simulink model "PC_MSFS_STATION"  (R2021b)
settings: Solver=FixedStepAuto  StartTime=0.0  StopTime=2000  FixedStep=0.03  RelTol=1e-3
undefined symbols (not defined in the file): CONTROL, DiscIntNeverNeededParam, f, MODEL, MODEL_INI
libraries: instrumentlib x22, SimConnectToolbox x3, simulink x2
(part 1 of 2)
settings Model: Creator=Andreas  LastModifiedBy=ae-dagbeyibor3
settings SolverCC: AlgebraicLoopSolver=TrustRegion
settings DebuggingCC: InheritedTsInSrcMsg=none  SFMachineParentedDataDiag=warning

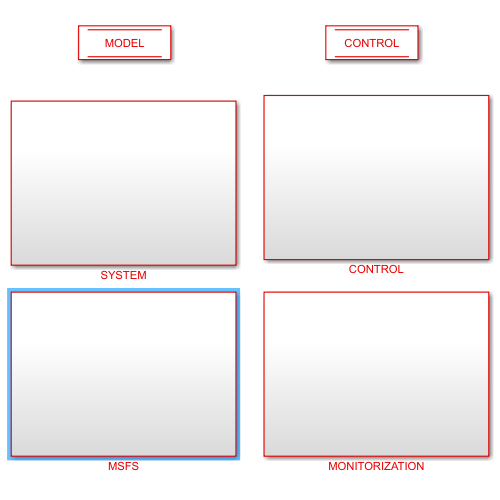
[thumbnail: Simulink's stored preview of the top-level diagram]
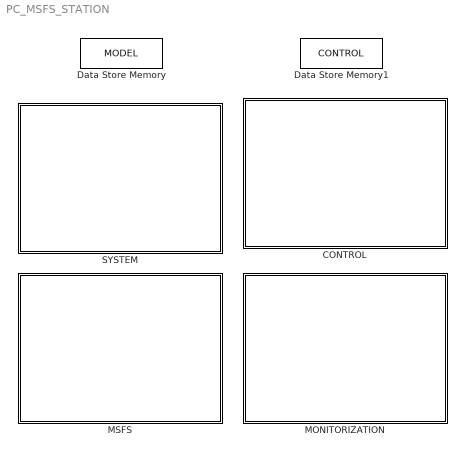
== system PC_MSFS_STATION ==
  CONTROL : Subsystem
  Data Store Memory : DataStoreMemory  DataStoreName=MODEL  ReadBeforeWriteMsg=warning  WriteAfterWriteMsg=warning  WriteAfterReadMsg=warning  InitialValue=MODEL_INI  ShowAdditionalParam=off  OutDataTypeStr=Bus: MODEL_Bus
  Data Store Memory1 : DataStoreMemory  DataStoreName=CONTROL  ReadBeforeWriteMsg=warning  WriteAfterWriteMsg=warning  WriteAfterReadMsg=warning  InitialValue=CONTROL_INI  ShowAdditionalParam=off  OutDataTypeStr=Bus: CONTROL_Bus
  MONITORIZATION : Subsystem
  MSFS : Subsystem
  SYSTEM : Subsystem

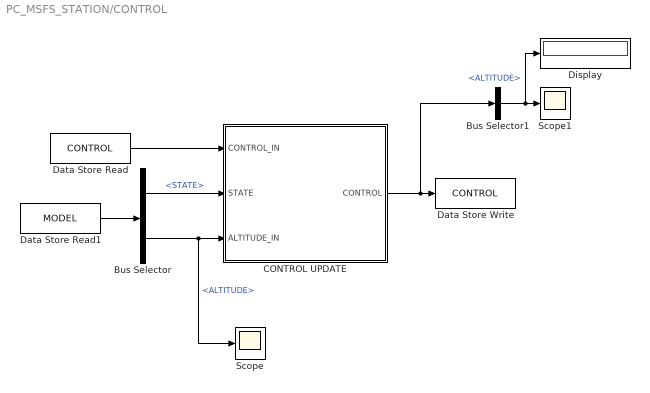
== system PC_MSFS_STATION/CONTROL ==
  Bus Selector : BusSelector  OutputSignals=STATE,INPUT.ALTITUDE
  Bus Selector1 : BusSelector  OutputSignals=PARAM.ALTITUDE
  CONTROL UPDATE : MATLAB Function  TreatAsAtomicUnit=on
  Data Store Read : DataStoreRead  DataStoreName=CONTROL  SampleTime=MODEL_INI.PARAM.SIM_SAMPLING_TIME  IndexOptions=Index vector (dialog)  Indices=1  OutputSizes=1
  Data Store Read1 : DataStoreRead  DataStoreName=MODEL  SampleTime=MODEL_INI.PARAM.SIM_SAMPLING_TIME  IndexOptions=Index vector (dialog)  Indices=1  OutputSizes=1
  Data Store Write : DataStoreWrite  DataStoreName=CONTROL  IndexOptions=Index vector (dialog)  Indices=1  OutputSizes=1
  Display : Display
  Scope : Scope
  Scope1 : Scope
  wires:
  Data Store Read/1 -> CONTROL UPDATE/1(CONTROL_IN)
  CONTROL UPDATE/1(CONTROL) -> Bus Selector1/1, Data Store Write/1
  Bus Selector/1 -> CONTROL UPDATE/2(STATE)  "<STATE>"
  Data Store Read1/1 -> Bus Selector/1
  Bus Selector/2 -> CONTROL UPDATE/3(ALTITUDE_IN), Scope/1  "<ALTITUDE>"
  Bus Selector1/1 -> Display/1, Scope1/1  "<ALTITUDE>"

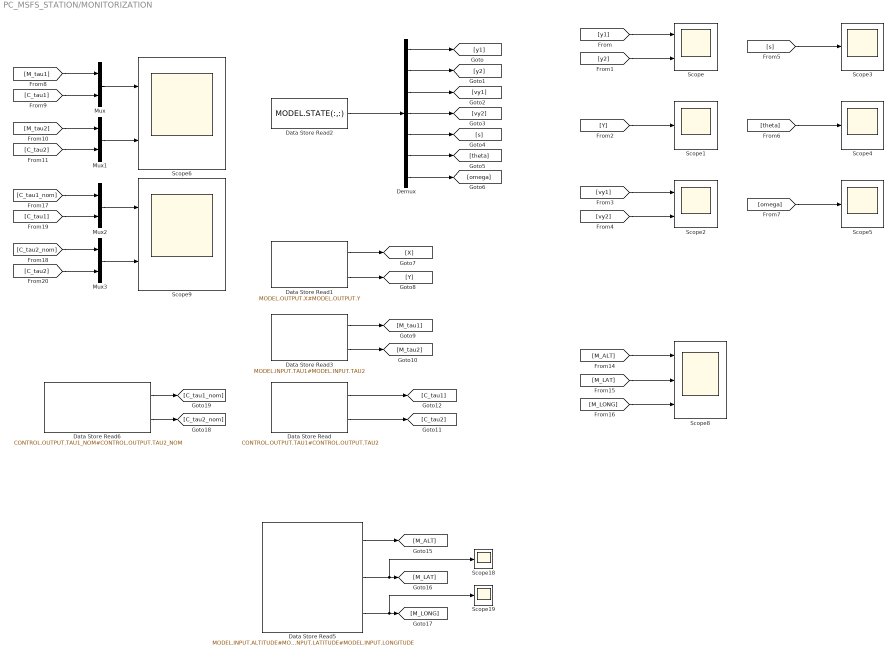
== system PC_MSFS_STATION/MONITORIZATION ==
  Data Store Read : DataStoreRead  DataStoreName=CONTROL  DataStoreElements=CONTROL.OUTPUT.TAU1#CONTROL.OUTPUT.TAU2  IndexOptions=Index vector (dialog)  Indices=1  OutputSizes=1
  Data Store Read1 : DataStoreRead  DataStoreName=MODEL  SampleTime=MODEL_INI.PARAM.SIM_SAMPLING_TIME  DataStoreElements=MODEL.OUTPUT.X#MODEL.OUTPUT.Y  IndexOptions=Index vector (dialog)  Indices=1  OutputSizes=1
  Data Store Read2 : DataStoreRead  DataStoreName=MODEL  SampleTime=MODEL_INI.PARAM.SIM_SAMPLING_TIME  DataStoreElements=MODEL.STATE(:,:)  IndexOptions=Index vector (dialog)  Indices=1  OutputSizes=1
  Data Store Read3 : DataStoreRead  DataStoreName=MODEL  SampleTime=MODEL_INI.PARAM.SIM_SAMPLING_TIME  DataStoreElements=MODEL.INPUT.TAU1#MODEL.INPUT.TAU2  IndexOptions=Index vector (dialog)  Indices=1  OutputSizes=1
  Data Store Read5 : DataStoreRead  DataStoreName=MODEL  SampleTime=MODEL_INI.PARAM.SIM_SAMPLING_TIME  DataStoreElements=MODEL.INPUT.ALTITUDE#MODEL.INPUT.LATITUDE#MODEL.INPUT.LONGITUDE  IndexOptions=Index vector (dialog)  Indices=1  OutputSizes=1
  Data Store Read6 : DataStoreRead  DataStoreName=CONTROL  DataStoreElements=CONTROL.OUTPUT.TAU1_NOM#CONTROL.OUTPUT.TAU2_NOM  IndexOptions=Index vector (dialog)  Indices=1  OutputSizes=1
  Demux : Demux  Outputs=7
  Mux{,1..3} (4 alike) : Mux  Inputs=2
  Scope{,2,6,9} (4 alike) : Scope  NumInputPorts=2
  Scope{1,3..5,18..19} (6 alike) : Scope
  Scope8 : Scope  NumInputPorts=3
  wires:
  Data Store Read2/1 -> Demux/1
  Demux/1 -> [y1]
  Demux/2 -> [y2]
  Demux/3 -> [vy1]
  Demux/4 -> [vy2]
  Demux/5 -> [s]
  Demux/6 -> [theta]
  Demux/7 -> [omega]
  [y1] -> Scope/1
  [y2] -> Scope/2
  Data Store Read1/1 -> [X]
  Data Store Read1/2 -> [Y]
  [Y] -> Scope1/1
  [vy2] -> Scope2/2
  [vy1] -> Scope2/1
  [s] -> Scope3/1
  [theta] -> Scope4/1
  [omega] -> Scope5/1
  Data Store Read3/1 -> [M_tau1]
  Data Store Read3/2 -> [M_tau2]
  Data Store Read/1 -> [C_tau1]
  Data Store Read/2 -> [C_tau2]
  Mux/1 -> Scope6/1
  Mux1/1 -> Scope6/2
  [M_tau1] -> Mux/1
  [M_tau2] -> Mux1/1
  [C_tau2] -> Mux1/2
  [C_tau1] -> Mux/2
  Data Store Read5/2 -> Scope18/1, [M_LAT]
  Data Store Read5/1 -> [M_ALT]
  Data Store Read5/3 -> Scope19/1, [M_LONG]
  [M_LAT] -> Scope8/2
  [M_ALT] -> Scope8/1
  [M_LONG] -> Scope8/3
  Data Store Read6/2 -> [C_tau2_nom]
  Data Store Read6/1 -> [C_tau1_nom]
  [C_tau1] -> Mux2/2
  [C_tau2] -> Mux3/2
  [C_tau2_nom] -> Mux3/1
  [C_tau1_nom] -> Mux2/1
  Mux3/1 -> Scope9/2
  Mux2/1 -> Scope9/1

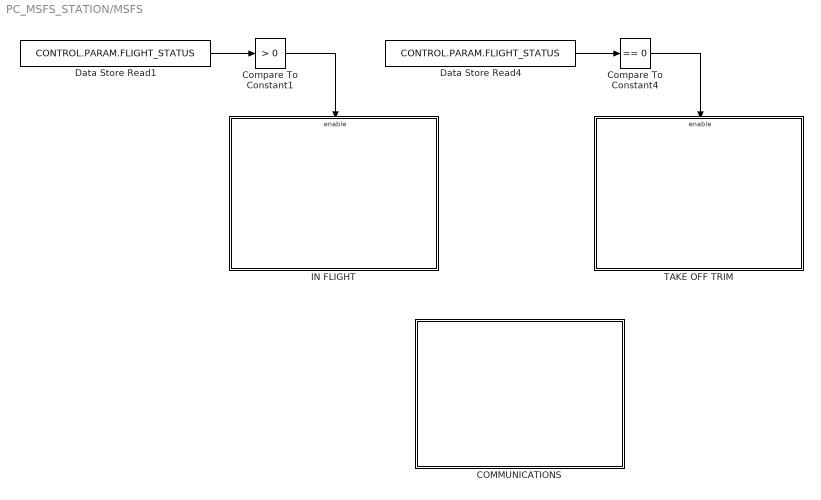
== system PC_MSFS_STATION/MSFS ==
  COMMUNICATIONS : Subsystem
  Compare To Constant1 : simulink/Logic and Bit Operations/Compare To Constant  relop=>  const=0  OutDataTypeStr=boolean
  Compare To Constant4 : simulink/Logic and Bit Operations/Compare To Constant  relop===  const=0  OutDataTypeStr=boolean
  Data Store Read1 : DataStoreRead  DataStoreName=CONTROL  DataStoreElements=CONTROL.PARAM.FLIGHT_STATUS  IndexOptions=Index vector (dialog)  Indices=1  OutputSizes=1
  Data Store Read4 : DataStoreRead  DataStoreName=CONTROL  DataStoreElements=CONTROL.PARAM.FLIGHT_STATUS  IndexOptions=Index vector (dialog)  Indices=1  OutputSizes=1
  IN FLIGHT : Subsystem
  TAKE OFF TRIM : Subsystem
  wires:
  Data Store Read1/1 -> Compare To Constant1/1
  Data Store Read4/1 -> Compare To Constant4/1
  Compare To Constant4/1 -> TAKE OFF TRIM/Enable
  Compare To Constant1/1 -> IN FLIGHT/Enable

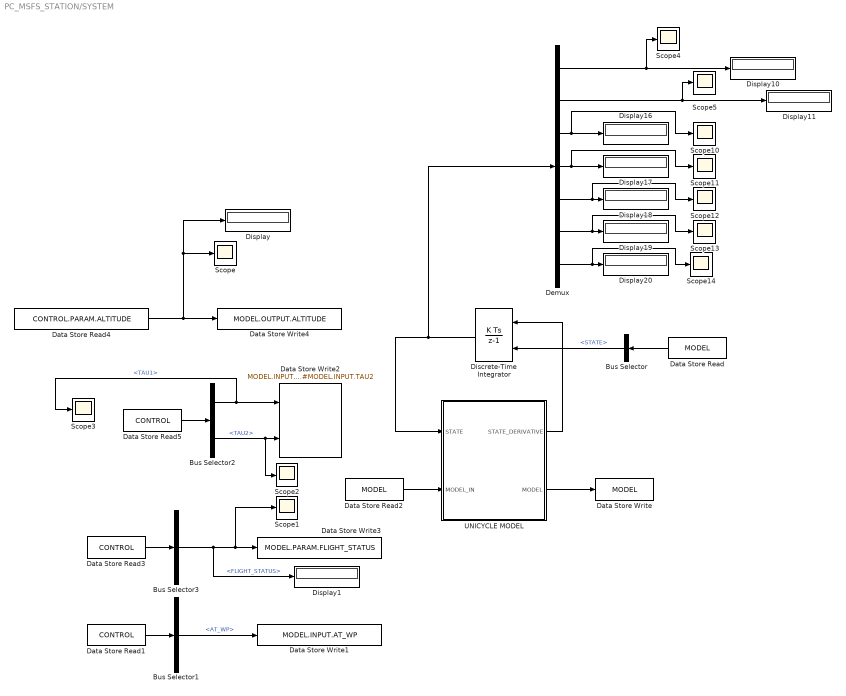
== system PC_MSFS_STATION/SYSTEM ==
  Bus Selector : BusSelector  OutputSignals=STATE
  Bus Selector1 : BusSelector  OutputSignals=OUTPUT.AT_WP
  Bus Selector2 : BusSelector  OutputSignals=OUTPUT.TAU1,OUTPUT.TAU2
  Bus Selector3 : BusSelector  OutputSignals=PARAM.FLIGHT_STATUS
  Data Store Read : DataStoreRead  DataStoreName=MODEL  SampleTime=MODEL_INI.PARAM.SIM_SAMPLING_TIME  IndexOptions=Index vector (dialog)  Indices=1  OutputSizes=1
  Data Store Read1 : DataStoreRead  DataStoreName=CONTROL  IndexOptions=Index vector (dialog)  Indices=1  OutputSizes=1
  Data Store Read2 : DataStoreRead  DataStoreName=MODEL  SampleTime=MODEL_INI.PARAM.SIM_SAMPLING_TIME  IndexOptions=Index vector (dialog)  Indices=1  OutputSizes=1
  Data Store Read3 : DataStoreRead  DataStoreName=CONTROL  IndexOptions=Index vector (dialog)  Indices=1  OutputSizes=1
  Data Store Read4 : DataStoreRead  DataStoreName=CONTROL  DataStoreElements=CONTROL.PARAM.ALTITUDE  IndexOptions=Index vector (dialog)  Indices=1  OutputSizes=1
  Data Store Read5 : DataStoreRead  DataStoreName=CONTROL  IndexOptions=Index vector (dialog)  Indices=1  OutputSizes=1
  Data Store Write : DataStoreWrite  DataStoreName=MODEL  IndexOptions=Index vector (dialog)  Indices=1  OutputSizes=1
  Data Store Write1 : DataStoreWrite  DataStoreName=MODEL  DataStoreElements=MODEL.INPUT.AT_WP  IndexOptions=Index vector (dialog)  Indices=1  OutputSizes=1
  Data Store Write2 : DataStoreWrite  DataStoreName=MODEL  DataStoreElements=MODEL.INPUT.TAU1#MODEL.INPUT.TAU2  IndexOptions=Index vector (dialog)  Indices=1  OutputSizes=1
  Data Store Write3 : DataStoreWrite  DataStoreName=MODEL  DataStoreElements=MODEL.PARAM.FLIGHT_STATUS  IndexOptions=Index vector (dialog)  Indices=1  OutputSizes=1
  Data Store Write4 : DataStoreWrite  DataStoreName=MODEL  DataStoreElements=MODEL.OUTPUT.ALTITUDE  IndexOptions=Index vector (dialog)  Indices=1  OutputSizes=1
  Demux : Demux  Outputs=7
  Discrete-Time Integrator : DiscreteIntegrator  InitialConditionSource=external  SampleTime=-1  ICPrevOutput=DiscIntNeverNeededParam  ICPrevScaledInput=DiscIntNeverNeededParam
  Display{,1,10..11,16..20} (9 alike) : Display
  Scope{,1..5,10..14} (11 alike) : Scope
  UNICYCLE MODEL : MATLAB Function  TreatAsAtomicUnit=on
  wires:
  Discrete-Time Integrator/1 -> Demux/1, UNICYCLE MODEL/1(STATE)
  UNICYCLE MODEL/1(STATE_DERIVATIVE) -> Discrete-Time Integrator/1
  Bus Selector/1 -> Discrete-Time Integrator/2  "<STATE>"
  Data Store Read/1 -> Bus Selector/1
  Data Store Read2/1 -> UNICYCLE MODEL/2(MODEL_IN)
  UNICYCLE MODEL/2(MODEL) -> Data Store Write/1
  Bus Selector2/2 -> Scope2/1, Data Store Write2/2  "<TAU2>"
  Bus Selector2/1 -> Scope3/1, Data Store Write2/1  "<TAU1>"
  Data Store Read5/1 -> Bus Selector2/1
  Data Store Read3/1 -> Bus Selector3/1
  Bus Selector3/1 -> Display1/1, Data Store Write3/1, Scope1/1  "<FLIGHT_STATUS>"
  Data Store Read4/1 -> Display/1, Scope/1, Data Store Write4/1
  Bus Selector1/1 -> Data Store Write1/1  "<AT_WP>"
  Data Store Read1/1 -> Bus Selector1/1
  Demux/1 -> Scope4/1, Display10/1
  Demux/2 -> Scope5/1, Display11/1
  Demux/6 -> Scope13/1, Display19/1
  Demux/3 -> Scope10/1, Display16/1
  Demux/4 -> Scope11/1, Display17/1
  Demux/5 -> Scope12/1, Display18/1
  Demux/7 -> Scope14/1, Display20/1

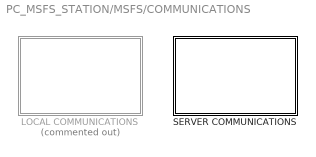
== system PC_MSFS_STATION/MSFS/COMMUNICATIONS ==
  LOCAL COMMUNICATIONS : Subsystem  Commented=on
  SERVER COMMUNICATIONS : Subsystem

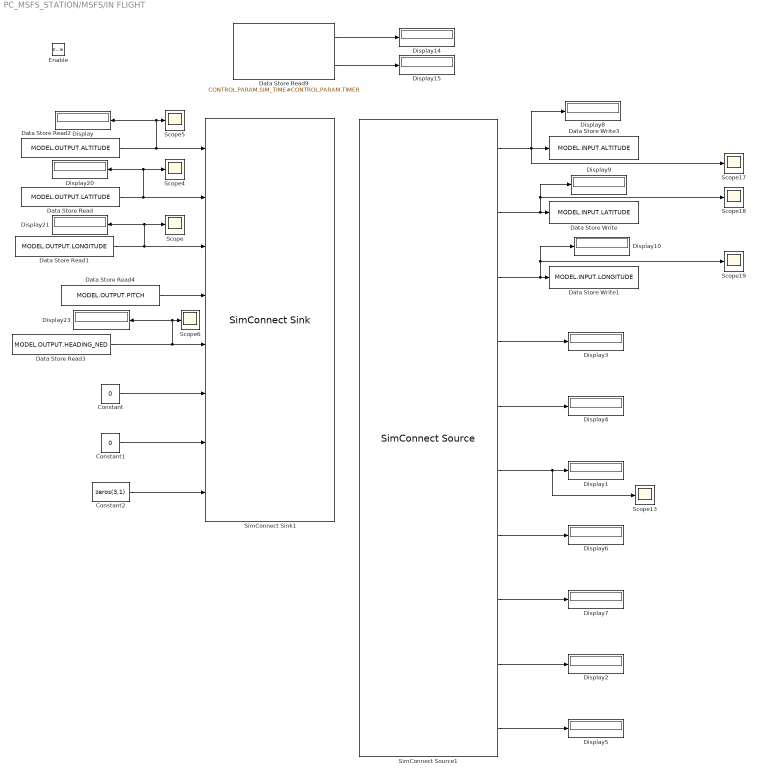
== system PC_MSFS_STATION/MSFS/IN FLIGHT ==
  Enable : EnablePort
  Constant : Constant  Value=0  SampleTime=-1
  Constant1 : Constant  Value=0  SampleTime=-1
  Constant2 : Constant  Value=zeros(3,1)  SampleTime=-1
  Data Store Read : DataStoreRead  DataStoreName=MODEL  DataStoreElements=MODEL.OUTPUT.LATITUDE  IndexOptions=Index vector (dialog)  Indices=1  OutputSizes=1
  Data Store Read1 : DataStoreRead  DataStoreName=MODEL  DataStoreElements=MODEL.OUTPUT.LONGITUDE  IndexOptions=Index vector (dialog)  Indices=1  OutputSizes=1
  Data Store Read2 : DataStoreRead  DataStoreName=MODEL  DataStoreElements=MODEL.OUTPUT.ALTITUDE  IndexOptions=Index vector (dialog)  Indices=1  OutputSizes=1
  Data Store Read3 : DataStoreRead  DataStoreName=MODEL  DataStoreElements=MODEL.OUTPUT.HEADING_NED  IndexOptions=Index vector (dialog)  Indices=1  OutputSizes=1
  Data Store Read4 : DataStoreRead  DataStoreName=MODEL  DataStoreElements=MODEL.OUTPUT.PITCH  IndexOptions=Index vector (dialog)  Indices=1  OutputSizes=1
  Data Store Read9 : DataStoreRead  DataStoreName=CONTROL  DataStoreElements=CONTROL.PARAM.SIM_TIME#CONTROL.PARAM.TIMER  IndexOptions=Index vector (dialog)  Indices=1  OutputSizes=1
  Data Store Write : DataStoreWrite  DataStoreName=MODEL  DataStoreElements=MODEL.INPUT.LATITUDE  IndexOptions=Index vector (dialog)  Indices=1  OutputSizes=1
  Data Store Write1 : DataStoreWrite  DataStoreName=MODEL  DataStoreElements=MODEL.INPUT.LONGITUDE  IndexOptions=Index vector (dialog)  Indices=1  OutputSizes=1
  Data Store Write3 : DataStoreWrite  DataStoreName=MODEL  DataStoreElements=MODEL.INPUT.ALTITUDE  IndexOptions=Index vector (dialog)  Indices=1  OutputSizes=1
  Display{,1..10,14..15,20..21,23} (16 alike) : Display
  Scope{,4..6,13,17..19} (8 alike) : Scope
  SimConnect Sink1 : SimConnectToolbox/SimConnect Sink  configurationIndex=0  connectionName=SimConnectSink  variables=|
      | PLANE ALTITUDE, FEET;
      | PLANE LATITUDE, RADIANS;
      | PLANE LONGITUDE, RADIANS;
      | PLANE PITCH DEGREES, RADIANS;
      | PLANE HEADING DEGREES TRUE, RADIANS;
      | PLANE BANK DEGREES, RADIANS;
      | AILERON POSITION, POSITION;
      | AILERON TRIM PCT, PERCENT;
      settings: SourceProductName=SimConnect Toolbox
      mask Display:
      | % This is a new mask on top of the base mask.
      | % Use "View base mask" link below to see the base mask.
      | %port_label('input', 1, 'Rudder Trim', 'texmode', 'on')
      | port_label('input', 1, 'PLANE ALTITUDE, FEET', 'texmode', 'on')
      | port_label('input', 2, 'PLANE LATITUDE, RADIANS', 'texmode', 'on')
      | port_label('input', 3, 'PLANE LONGITUDE, RADIANS', 'texmode', 'on')
      | port_label('input', 4, 'PITCH DEGREES, RADIANS', 'texmode', 'on')
      | port_label('input', 5, 'HEADING DEGREES TRUE, RADIANS', 'texmode', 'on')
      | port_label('input', 6, 'PLANE BANK DEGREES, RADIANS;', 'texmode', 'on')
      | port_label('input', 7, 'AILERON POSITION, POSITION', 'texmode', 'on')
      | port_label('input', 8, 'AILERON TRIM PCT, PERCENT OVER 100', 'texmode', 'on')
  SimConnect Source1 : SimConnectToolbox/SimConnect Source  configurationIndex=0  connectionName=SimConnectSource  variables=|
      | PLANE ALTITUDE, FEET;
      | PLANE LATITUDE, RADIANS;
      | PLANE LONGITUDE, RADIANS;
      | ROTATION VELOCITY BODY X, FEET PER SECOND;
      | PLANE PITCH DEGREES, RADIANS;
      | PLANE HEADING DEGREES TRUE, RADIANS;
      | PLANE HEADING DEGREES MAGNETIC, RADIANS;
      | PLANE HEADING DEGREES GYRO, DEGREES;
      | AILERON POSITION, POSITION;
      | AILERON TRIM PCT, PERCENT OVER 100;
      settings: SourceProductName=SimConnect Toolbox
      mask Display:
      | % This is a new mask on top of the base mask.
      | % Use "View base mask" link below to see the base mask.
      | % port_label('output', 1, 'g', 'texmode', 'on')
      | port_label('output', 1, 'PLANE ALTITUDE, FEET', 'texmode', 'on')
      | port_label('output', 2, 'PLANE LATITUDE, RADIANS', 'texmode', 'on')
      | port_label('output', 3, 'PLANE LONGITUDE, RADIANS', 'texmode', 'on')
      | port_label('output', 4, 'VELOCITY BODY X, FEET PER SECOND', 'texmode', 'on')
      | port_label('output', 5, 'PITCH DEGREES, RADIANS', 'texmode', 'on')
      | port_label('output', 6, 'HEADING DEGREES TRUE, RADIANS', 'texmode', 'on')
      | port_label('output', 7, 'HEADING DEGREES MAGNETIC, RADIANS', 'texmode', 'on')
      | port_label('output', 8, 'HEADING DEGREES GYRO, DEGREES', 'texmode', 'on')
      | port_label('output', 9, 'AILERON POSITION, POSITION', 'texmode', 'on')
      | port_label('output', 10, 'AILERON TRIM PCT, PERCENT OVER 100', 'texmode', 'on')
  wires:
  Constant2/1 -> SimConnect Sink1/8
  SimConnect Source1/9 -> Display2/1
  Constant/1 -> SimConnect Sink1/6
  Data Store Read1/1 -> Display21/1, Scope/1, SimConnect Sink1/3
  Constant1/1 -> SimConnect Sink1/7
  SimConnect Source1/5 -> Display4/1
  SimConnect Source1/3 -> Display10/1, Scope19/1, Data Store Write1/1
  SimConnect Source1/2 -> Display9/1, Scope18/1, Data Store Write/1
  SimConnect Source1/8 -> Display7/1
  SimConnect Source1/6 -> Scope13/1, Display1/1
  Data Store Read2/1 -> Display/1, Scope5/1, SimConnect Sink1/1
  Data Store Read/1 -> Display20/1, Scope4/1, SimConnect Sink1/2
  Data Store Read4/1 -> SimConnect Sink1/4
  SimConnect Source1/4 -> Display3/1
  SimConnect Source1/1 -> Data Store Write3/1, Display8/1, Scope17/1
  SimConnect Source1/7 -> Display6/1
  SimConnect Source1/10 -> Display5/1
  Data Store Read9/1 -> Display14/1
  Data Store Read9/2 -> Display15/1
  Data Store Read3/1 -> Display23/1, Scope6/1, SimConnect Sink1/5

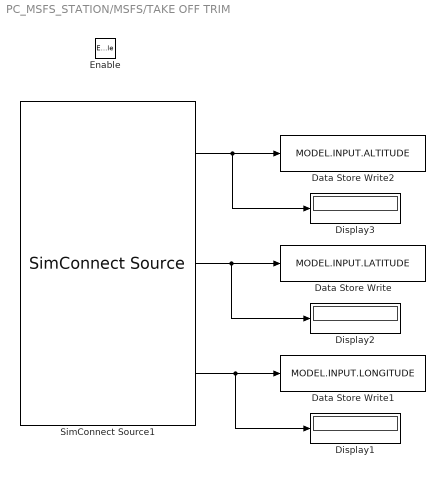
== system PC_MSFS_STATION/MSFS/TAKE OFF TRIM ==
  Enable : EnablePort
  Data Store Write : DataStoreWrite  DataStoreName=MODEL  DataStoreElements=MODEL.INPUT.LATITUDE  IndexOptions=Index vector (dialog)  Indices=1  OutputSizes=1
  Data Store Write1 : DataStoreWrite  DataStoreName=MODEL  DataStoreElements=MODEL.INPUT.LONGITUDE  IndexOptions=Index vector (dialog)  Indices=1  OutputSizes=1
  Data Store Write2 : DataStoreWrite  DataStoreName=MODEL  DataStoreElements=MODEL.INPUT.ALTITUDE  IndexOptions=Index vector (dialog)  Indices=1  OutputSizes=1
  Display1 : Display
  Display2 : Display
  Display3 : Display
  SimConnect Source1 : SimConnectToolbox/SimConnect Source  configurationIndex=0  connectionName=SimConnectSource  variables=|
      | PLANE ALTITUDE, FEET;
      | PLANE LATITUDE, RADIANS;
      | PLANE LONGITUDE, RADIANS;
      settings: SourceProductName=SimConnect Toolbox
      mask Display:
      | % This is a new mask on top of the base mask.
      | % Use "View base mask" link below to see the base mask.
      | % port_label('output', 1, 'g', 'texmode', 'on')
      | port_label('output', 1, 'PLANE ALTITUDE, FEET', 'texmode', 'on')
      | port_label('output', 2, 'PLANE LATITUDE, RADIANS', 'texmode', 'on')
      | port_label('output', 3, 'PLANE LONGITUDE, RADIANS', 'texmode', 'on')
  wires:
  SimConnect Source1/2 -> Data Store Write/1, Display2/1
  SimConnect Source1/1 -> Display3/1, Data Store Write2/1
  SimConnect Source1/3 -> Display1/1, Data Store Write1/1

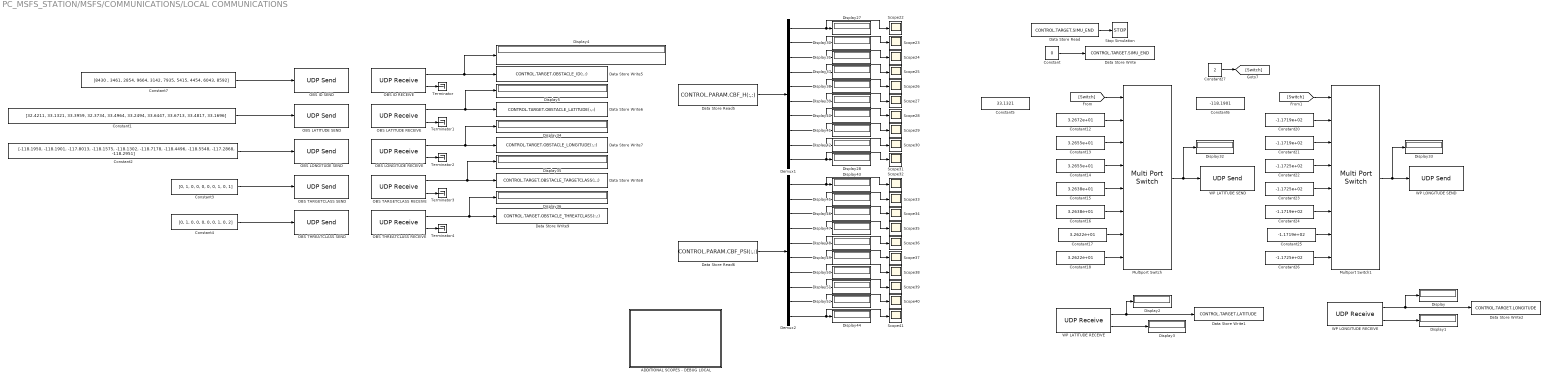
== system PC_MSFS_STATION/MSFS/COMMUNICATIONS/LOCAL COMMUNICATIONS ==
  ADDITIONAL SCOPES - DEBUG LOCAL : Subsystem
  Constant : Constant  Value=0  SampleTime=-1
  Constant1 : Constant  Value=[32.4211, 33.1321, 33.3959, 32.3734, 33.4964, 33.2494, 33.6447, 33.6713, 33.4817, 33.1696]  SampleTime=-1
  Constant12 : Constant  Value=3.2672e+01  SampleTime=0.03
  Constant13 : Constant  Value=3.2655e+01  SampleTime=0.03
  Constant14 : Constant  Value=3.2655e+01  SampleTime=0.03
  Constant15 : Constant  Value=3.2638e+01  SampleTime=0.03
  Constant16 : Constant  Value=3.2638e+01  SampleTime=0.03
  Constant17 : Constant  Value=3.2622e+01  SampleTime=0.03
  Constant18 : Constant  Value=3.2622e+01  SampleTime=0.03
  Constant2 : Constant  Value=[-118.1950, -118.1901, -117.8013, -118.1575, -118.1302, -118.7178, -118.4496, -118.5548, -117.2868, -118.2951]  SampleTime=-1
  Constant{20..21,24..25} (4 alike) : Constant  Value=-1.1719e+02  SampleTime=0.03
  Constant22 : Constant  Value=-1.1725e+02  SampleTime=0.03
  Constant23 : Constant  Value=-1.1725e+02  SampleTime=0.03
  Constant26 : Constant  Value=-1.1725e+02  SampleTime=0.03
  Constant27 : Constant  Value=2  SampleTime=-1
  Constant3 : Constant  Value=[0, 1, 0, 0, 0, 0, 0, 1, 0, 1]  SampleTime=-1
  Constant4 : Constant  Value=[0, 1, 0, 0, 0, 0, 0, 1, 0, 2]  SampleTime=-1
  Constant5 : Constant  Value=33.1321  SampleTime=0.03
  Constant6 : Constant  Value=-118.1901  SampleTime=0.03
  Constant7 : Constant  Value=[8430 , 3461, 2854, 9664, 3142, 7935, 5415, 4454, 6043, 8592]  SampleTime=-1
  Data Store Read : DataStoreRead  DataStoreName=CONTROL  DataStoreElements=CONTROL.TARGET.SIMU_END  IndexOptions=Index vector (dialog)  Indices=1  OutputSizes=1
  Data Store Read5 : DataStoreRead  DataStoreName=CONTROL  DataStoreElements=CONTROL.PARAM.CBF_H(:,:)  IndexOptions=Index vector (dialog)  Indices=1  OutputSizes=1
  Data Store Read6 : DataStoreRead  DataStoreName=CONTROL  DataStoreElements=CONTROL.PARAM.CBF_PSI(:,:)  IndexOptions=Index vector (dialog)  Indices=1  OutputSizes=1
  Data Store Write : DataStoreWrite  DataStoreName=CONTROL  DataStoreElements=CONTROL.TARGET.SIMU_END  IndexOptions=Index vector (dialog)  Indices=1  OutputSizes=1
  Data Store Write1 : DataStoreWrite  DataStoreName=CONTROL  DataStoreElements=CONTROL.TARGET.LATITUDE  IndexOptions=Index vector (dialog)  Indices=1  OutputSizes=1
  Data Store Write2 : DataStoreWrite  DataStoreName=CONTROL  DataStoreElements=CONTROL.TARGET.LONGITUDE  IndexOptions=Index vector (dialog)  Indices=1  OutputSizes=1
  Data Store Write5 : DataStoreWrite  DataStoreName=CONTROL  DataStoreElements=CONTROL.TARGET.OBSTACLE_ID(:,:)  IndexOptions=Index vector (dialog)  Indices=1  OutputSizes=1
  Data Store Write6 : DataStoreWrite  DataStoreName=CONTROL  DataStoreElements=CONTROL.TARGET.OBSTACLE_LATITUDE(:,:)  IndexOptions=Index vector (dialog)  Indices=1  OutputSizes=1
  Data Store Write7 : DataStoreWrite  DataStoreName=CONTROL  DataStoreElements=CONTROL.TARGET.OBSTACLE_LONGITUDE(:,:)  IndexOptions=Index vector (dialog)  Indices=1  OutputSizes=1
  Data Store Write8 : DataStoreWrite  DataStoreName=CONTROL  DataStoreElements=CONTROL.TARGET.OBSTACLE_TARGETCLASS(:,:)  IndexOptions=Index vector (dialog)  Indices=1  OutputSizes=1
  Data Store Write9 : DataStoreWrite  DataStoreName=CONTROL  DataStoreElements=CONTROL.TARGET.OBSTACLE_THREATCLASS(:,:)  IndexOptions=Index vector (dialog)  Indices=1  OutputSizes=1
  Demux1 : Demux  Outputs=10
  Demux2 : Demux  Outputs=10
  Display{,1..5,27..28,30..52} (31 alike) : Display
  Multiport Switch : MultiPortSwitch  Inputs=7
  Multiport Switch1 : MultiPortSwitch  Inputs=7
  OBS ID RECEIVE : instrumentlib/UDP Receive  Host=127.0.0.1  Port=8081  LocalPort=8082  EnablePortSharing=off  GetLatestData=off  DataSize="[10   1]"  DataType=double  ASCIIFormatting=%f,  Terminator=LF  ByteOrder=BigEndian  EnableBlockingMode=off  Timeout=10  SampleTime=-1  LocalAddress=127.0.0.1
  OBS ID SEND : instrumentlib/UDP Send  Host=127.0.0.1  Port=8082  LocalPort=8081  EnablePortSharing=off  ByteOrder=BigEndian  OutputDatagramPacketSize=512  EnableBlockingMode=on  LocalAddress=127.0.0.1
  OBS LATITUDE RECEIVE : instrumentlib/UDP Receive  Host=127.0.0.1  Port=8083  LocalPort=8084  EnablePortSharing=off  GetLatestData=off  DataSize="[10   1]"  DataType=double  ASCIIFormatting=%f,  Terminator=LF  ByteOrder=BigEndian  EnableBlockingMode=off  Timeout=10  SampleTime=-1  LocalAddress=127.0.0.1
  OBS LATITUDE SEND : instrumentlib/UDP Send  Host=127.0.0.1  Port=8084  LocalPort=8083  EnablePortSharing=off  ByteOrder=BigEndian  OutputDatagramPacketSize=512  EnableBlockingMode=on  LocalAddress=127.0.0.1
  OBS LONGITUDE RECEIVE : instrumentlib/UDP Receive  Host=127.0.0.1  Port=8085  LocalPort=8086  EnablePortSharing=off  GetLatestData=off  DataSize="[10   1]"  DataType=double  ASCIIFormatting=%f,  Terminator=LF  ByteOrder=BigEndian  EnableBlockingMode=off  Timeout=10  SampleTime=-1  LocalAddress=127.0.0.1
  OBS LONGITUDE SEND : instrumentlib/UDP Send  Host=127.0.0.1  Port=8086  LocalPort=8085  EnablePortSharing=off  ByteOrder=BigEndian  OutputDatagramPacketSize=512  EnableBlockingMode=on  LocalAddress=127.0.0.1
  OBS TARGETCLASS RECEIVE : instrumentlib/UDP Receive  Host=127.0.0.1  Port=7087  LocalPort=7088  EnablePortSharing=off  GetLatestData=off  DataSize="[10   1]"  DataType=double  ASCIIFormatting=%f,  Terminator=LF  ByteOrder=BigEndian  EnableBlockingMode=off  Timeout=10  SampleTime=-1  LocalAddress=127.0.0.1
  OBS TARGETCLASS SEND : instrumentlib/UDP Send  Host=127.0.0.1  Port=7088  LocalPort=7087  EnablePortSharing=off  ByteOrder=BigEndian  OutputDatagramPacketSize=512  EnableBlockingMode=on  LocalAddress=127.0.0.1
  OBS THREATCLASS RECEIVE : instrumentlib/UDP Receive  Host=127.0.0.1  Port=7089  LocalPort=7080  EnablePortSharing=off  GetLatestData=off  DataSize="[10   1]"  DataType=double  ASCIIFormatting=%f,  Terminator=LF  ByteOrder=BigEndian  EnableBlockingMode=off  Timeout=10  SampleTime=-1  LocalAddress=127.0.0.1
  OBS THREATCLASS SEND : instrumentlib/UDP Send  Host=127.0.0.1  Port=7080  LocalPort=7089  EnablePortSharing=off  ByteOrder=BigEndian  OutputDatagramPacketSize=512  EnableBlockingMode=on  LocalAddress=127.0.0.1
  Scope{22..41} (20 alike) : Scope
  Stop Simulation : Stop
  Terminator{,1..4} (5 alike) : Terminator
  WP LATITUDE RECEIVE : instrumentlib/UDP Receive  Host=127.0.0.1  Port=8087  LocalPort=8080  EnablePortSharing=off  GetLatestData=off  DataSize=[1 1]  DataType=double  ASCIIFormatting=%f,  Terminator=LF  ByteOrder=BigEndian  EnableBlockingMode=off  Timeout=10  SampleTime=-1  LocalAddress=127.0.0.1
  WP LATITUDE SEND : instrumentlib/UDP Send  Host=127.0.0.1  Port=8080  LocalPort=8087  EnablePortSharing=off  ByteOrder=BigEndian  OutputDatagramPacketSize=512  EnableBlockingMode=on  LocalAddress=127.0.0.1
  WP LONGITUDE RECEIVE : instrumentlib/UDP Receive  Host=127.0.0.1  Port=8089  LocalPort=8088  EnablePortSharing=off  GetLatestData=off  DataSize=[1 1]  DataType=double  ASCIIFormatting=%f,  Terminator=LF  ByteOrder=BigEndian  EnableBlockingMode=off  Timeout=10  SampleTime=-1  LocalAddress=127.0.0.1
  WP LONGITUDE SEND : instrumentlib/UDP Send  Host=127.0.0.1  Port=8088  LocalPort=8089  EnablePortSharing=off  ByteOrder=BigEndian  OutputDatagramPacketSize=512  EnableBlockingMode=on  LocalAddress=127.0.0.1
  wires:
  WP LATITUDE RECEIVE/2 -> Display3/1
  WP LATITUDE RECEIVE/1 -> Display2/1, Data Store Write1/1
  WP LONGITUDE RECEIVE/1 -> Data Store Write2/1, Display/1
  WP LONGITUDE RECEIVE/2 -> Display1/1
  Data Store Read/1 -> Stop Simulation/1
  Constant/1 -> Data Store Write/1
  [Switch] -> Multiport Switch/1
  Constant13/1 -> Multiport Switch/3
  Constant14/1 -> Multiport Switch/4
  Constant15/1 -> Multiport Switch/5
  Constant16/1 -> Multiport Switch/6
  Constant17/1 -> Multiport Switch/7
  Constant18/1 -> Multiport Switch/8
  Multiport Switch/1 -> WP LATITUDE SEND/1, Display32/1
  Multiport Switch1/1 -> WP LONGITUDE SEND/1, Display33/1
  Constant26/1 -> Multiport Switch1/8
  Constant25/1 -> Multiport Switch1/7
  Constant24/1 -> Multiport Switch1/6
  Constant23/1 -> Multiport Switch1/5
  Constant22/1 -> Multiport Switch1/4
  Constant21/1 -> Multiport Switch1/3
  [Switch] -> Multiport Switch1/1
  Constant27/1 -> [Switch]
  OBS ID RECEIVE/1 -> Data Store Write5/1, Display4/1
  OBS LATITUDE RECEIVE/1 -> Data Store Write6/1, Display5/1
  OBS LONGITUDE RECEIVE/1 -> Data Store Write7/1, Display34/1
  OBS TARGETCLASS RECEIVE/1 -> Display35/1, Data Store Write8/1
  OBS THREATCLASS RECEIVE/1 -> Display36/1, Data Store Write9/1
  OBS ID RECEIVE/2 -> Terminator/1
  OBS LATITUDE RECEIVE/2 -> Terminator1/1
  OBS LONGITUDE RECEIVE/2 -> Terminator2/1
  OBS TARGETCLASS RECEIVE/2 -> Terminator3/1
  OBS THREATCLASS RECEIVE/2 -> Terminator4/1
  Constant7/1 -> OBS ID SEND/1
  Constant1/1 -> OBS LATITUDE SEND/1
  Constant2/1 -> OBS LONGITUDE SEND/1
  Constant4/1 -> OBS THREATCLASS SEND/1
  Data Store Read5/1 -> Demux1/1
  Demux1/1 -> Scope22/1, Display27/1
  Demux1/2 -> Scope23/1, Display30/1
  Demux1/3 -> Scope24/1, Display31/1
  Demux1/4 -> Scope25/1, Display37/1
  Demux1/5 -> Scope26/1, Display38/1
  Demux1/6 -> Scope27/1, Display39/1
  Demux1/7 -> Scope28/1, Display40/1
  Demux1/8 -> Scope29/1, Display41/1
  Demux1/9 -> Scope30/1, Display42/1
  Demux1/10 -> Scope31/1, Display28/1
  Demux2/10 -> Display44/1, Scope41/1
  Demux2/9 -> Display52/1, Scope40/1
  Demux2/8 -> Display51/1, Scope39/1
  Demux2/7 -> Display50/1, Scope38/1
  Demux2/6 -> Display49/1, Scope37/1
  Demux2/5 -> Display48/1, Scope36/1
  Demux2/4 -> Display47/1, Scope35/1
  Demux2/3 -> Display46/1, Scope34/1
  Demux2/2 -> Display45/1, Scope33/1
  Demux2/1 -> Display43/1, Scope32/1
  Data Store Read6/1 -> Demux2/1
  Constant12/1 -> Multiport Switch/2
  Constant20/1 -> Multiport Switch1/2
  Constant3/1 -> OBS TARGETCLASS SEND/1

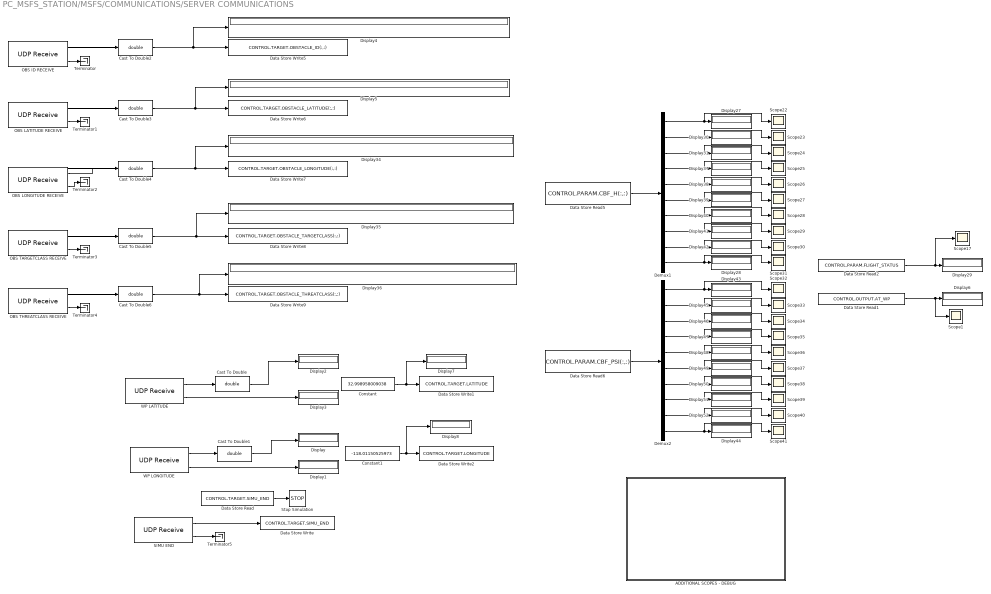
== system PC_MSFS_STATION/MSFS/COMMUNICATIONS/SERVER COMMUNICATIONS ==
  ADDITIONAL SCOPES - DEBUG : Subsystem
  Cast To Double{,1..6} (7 alike) : DataTypeConversion  OutDataTypeStr=double
  Constant : Constant  Value=32.998958009038  SampleTime=-1
  Constant1 : Constant  Value=-118.01150525973  SampleTime=-1
  Data Store Read : DataStoreRead  DataStoreName=CONTROL  DataStoreElements=CONTROL.TARGET.SIMU_END  IndexOptions=Index vector (dialog)  Indices=1  OutputSizes=1
  Data Store Read1 : DataStoreRead  DataStoreName=CONTROL  DataStoreElements=CONTROL.OUTPUT.AT_WP  IndexOptions=Index vector (dialog)  Indices=1  OutputSizes=1
  Data Store Read2 : DataStoreRead  DataStoreName=CONTROL  DataStoreElements=CONTROL.PARAM.FLIGHT_STATUS  IndexOptions=Index vector (dialog)  Indices=1  OutputSizes=1
  Data Store Read5 : DataStoreRead  DataStoreName=CONTROL  DataStoreElements=CONTROL.PARAM.CBF_H(:,:)  IndexOptions=Index vector (dialog)  Indices=1  OutputSizes=1
  Data Store Read6 : DataStoreRead  DataStoreName=CONTROL  DataStoreElements=CONTROL.PARAM.CBF_PSI(:,:)  IndexOptions=Index vector (dialog)  Indices=1  OutputSizes=1
  Data Store Write : DataStoreWrite  DataStoreName=CONTROL  DataStoreElements=CONTROL.TARGET.SIMU_END  IndexOptions=Index vector (dialog)  Indices=1  OutputSizes=1
  Data Store Write1 : DataStoreWrite  DataStoreName=CONTROL  DataStoreElements=CONTROL.TARGET.LATITUDE  IndexOptions=Index vector (dialog)  Indices=1  OutputSizes=1
  Data Store Write2 : DataStoreWrite  DataStoreName=CONTROL  DataStoreElements=CONTROL.TARGET.LONGITUDE  IndexOptions=Index vector (dialog)  Indices=1  OutputSizes=1
  Data Store Write5 : DataStoreWrite  DataStoreName=CONTROL  DataStoreElements=CONTROL.TARGET.OBSTACLE_ID(:,:)  IndexOptions=Index vector (dialog)  Indices=1  OutputSizes=1
  Data Store Write6 : DataStoreWrite  DataStoreName=CONTROL  DataStoreElements=CONTROL.TARGET.OBSTACLE_LATITUDE(:,:)  IndexOptions=Index vector (dialog)  Indices=1  OutputSizes=1
  Data Store Write7 : DataStoreWrite  DataStoreName=CONTROL  DataStoreElements=CONTROL.TARGET.OBSTACLE_LONGITUDE(:,:)  IndexOptions=Index vector (dialog)  Indices=1  OutputSizes=1
  Data Store Write8 : DataStoreWrite  DataStoreName=CONTROL  DataStoreElements=CONTROL.TARGET.OBSTACLE_TARGETCLASS(:,:)  IndexOptions=Index vector (dialog)  Indices=1  OutputSizes=1
  Data Store Write9 : DataStoreWrite  DataStoreName=CONTROL  DataStoreElements=CONTROL.TARGET.OBSTACLE_THREATCLASS(:,:)  IndexOptions=Index vector (dialog)  Indices=1  OutputSizes=1
  Demux1 : Demux  Outputs=10
  Demux2 : Demux  Outputs=10
  Display{,1..8,27..31,34..52} (33 alike) : Display
  OBS ID RECEIVE : instrumentlib/UDP Receive  Host=127.0.0.1  Port=8081  LocalPort=8082  EnablePortSharing=off  GetLatestData=off  DataSize="[10   1]"  DataType=double  ASCIIFormatting=%f,  Terminator=LF  ByteOrder=BigEndian  EnableBlockingMode=off  Timeout=10  SampleTime=-1  LocalAddress=127.0.0.1
  OBS LATITUDE RECEIVE : instrumentlib/UDP Receive  Host=127.0.0.1  Port=8083  LocalPort=8084  EnablePortSharing=off  GetLatestData=off  DataSize="[10   1]"  DataType=double  ASCIIFormatting=%f,  Terminator=LF  ByteOrder=BigEndian  EnableBlockingMode=off  Timeout=10  SampleTime=-1  LocalAddress=127.0.0.1
  OBS LONGITUDE RECEIVE : instrumentlib/UDP Receive  Host=127.0.0.1  Port=8085  LocalPort=8086  EnablePortSharing=off  GetLatestData=off  DataSize="[10   1]"  DataType=double  ASCIIFormatting=%f,  Terminator=LF  ByteOrder=BigEndian  EnableBlockingMode=off  Timeout=10  SampleTime=-1  LocalAddress=127.0.0.1
  OBS TARGETCLASS RECEIVE : instrumentlib/UDP Receive  Host=127.0.0.1  Port=7087  LocalPort=7088  EnablePortSharing=off  GetLatestData=off  DataSize="[10   1]"  DataType=double  ASCIIFormatting=%f,  Terminator=LF  ByteOrder=BigEndian  EnableBlockingMode=off  Timeout=10  SampleTime=-1  LocalAddress=127.0.0.1
  OBS THREATCLASS RECEIVE : instrumentlib/UDP Receive  Host=127.0.0.1  Port=7089  LocalPort=7080  EnablePortSharing=off  GetLatestData=off  DataSize="[10   1]"  DataType=double  ASCIIFormatting=%f,  Terminator=LF  ByteOrder=BigEndian  EnableBlockingMode=off  Timeout=10  SampleTime=-1  LocalAddress=127.0.0.1
  SIMU END : instrumentlib/UDP Receive  Host=127.0.0.1  Port=7086  LocalPort=7084  EnablePortSharing=off  GetLatestData=off  DataSize=[1 1]  DataType=double  ASCIIFormatting=%f,  Terminator=LF  ByteOrder=BigEndian  EnableBlockingMode=off  Timeout=10  SampleTime=-1  LocalAddress=127.0.0.1
  Scope{1,17,22..41} (22 alike) : Scope
  Stop Simulation : Stop
  Terminator{,1..5} (6 alike) : Terminator
  WP LATITUDE : instrumentlib/UDP Receive  Host=127.0.0.1  Port=8081  LocalPort=8080  EnablePortSharing=off  GetLatestData=off  DataSize=[1 1]  DataType=single  ASCIIFormatting=%f,  Terminator=LF  ByteOrder=BigEndian  EnableBlockingMode=off  Timeout=10  SampleTime=-1  LocalAddress=127.0.0.1
  WP LONGITUDE : instrumentlib/UDP Receive  Host=127.0.0.1  Port=8081  LocalPort=8088  EnablePortSharing=off  GetLatestData=off  DataSize=[1 1]  DataType=single  ASCIIFormatting=%f,  Terminator=LF  ByteOrder=BigEndian  EnableBlockingMode=off  Timeout=10  SampleTime=-1  LocalAddress=127.0.0.1
  wires:
  WP LONGITUDE/2 -> Display1/1
  Data Store Read1/1 -> Display6/1, Scope1/1
  Data Store Read2/1 -> Display29/1, Scope17/1
  WP LATITUDE/2 -> Display3/1
  WP LATITUDE/1 -> Cast To Double/1
  Cast To Double/1 -> Display2/1
  WP LONGITUDE/1 -> Cast To Double1/1
  Cast To Double1/1 -> Display/1
  Demux1/4 -> Scope25/1, Display37/1
  Demux1/2 -> Scope23/1, Display30/1
  Data Store Read6/1 -> Demux2/1
  Demux2/1 -> Display43/1, Scope32/1
  Demux2/3 -> Display46/1, Scope34/1
  Demux2/2 -> Display45/1, Scope33/1
  Demux2/7 -> Display50/1, Scope38/1
  Demux2/8 -> Display51/1, Scope39/1
  Demux2/9 -> Display52/1, Scope40/1
  Demux2/10 -> Display44/1, Scope41/1
  Demux2/6 -> Display49/1, Scope37/1
  Demux1/7 -> Scope28/1, Display40/1
  Demux2/4 -> Display47/1, Scope35/1
  Demux2/5 -> Display48/1, Scope36/1
  OBS ID RECEIVE/1 -> Cast To Double2/1
  Demux1/6 -> Scope27/1, Display39/1
  OBS LATITUDE RECEIVE/1 -> Cast To Double3/1
  Demux1/5 -> Scope26/1, Display38/1
  OBS THREATCLASS RECEIVE/1 -> Cast To Double6/1
  Demux1/9 -> Scope30/1, Display42/1
  OBS TARGETCLASS RECEIVE/2 -> Terminator3/1
  Demux1/8 -> Scope29/1, Display41/1
  OBS LONGITUDE RECEIVE/2 -> Terminator2/1
  OBS LATITUDE RECEIVE/2 -> Terminator1/1
  OBS ID RECEIVE/2 -> Terminator/1
  Demux1/1 -> Scope22/1, Display27/1
  OBS LONGITUDE RECEIVE/1 -> Cast To Double4/1
  Demux1/3 -> Scope24/1, Display31/1
  OBS TARGETCLASS RECEIVE/1 -> Cast To Double5/1
  OBS THREATCLASS RECEIVE/2 -> Terminator4/1
  Demux1/10 -> Scope31/1, Display28/1
  Data Store Read5/1 -> Demux1/1
  Cast To Double2/1 -> Data Store Write5/1, Display4/1
  Cast To Double3/1 -> Data Store Write6/1, Display5/1
  Cast To Double4/1 -> Data Store Write7/1, Display34/1
  Cast To Double5/1 -> Display35/1, Data Store Write8/1
  Cast To Double6/1 -> Display36/1, Data Store Write9/1
  Data Store Read/1 -> Stop Simulation/1
  SIMU END/2 -> Terminator5/1
  SIMU END/1 -> Data Store Write/1
  Constant/1 -> Display7/1, Data Store Write1/1
  Constant1/1 -> Display8/1, Data Store Write2/1

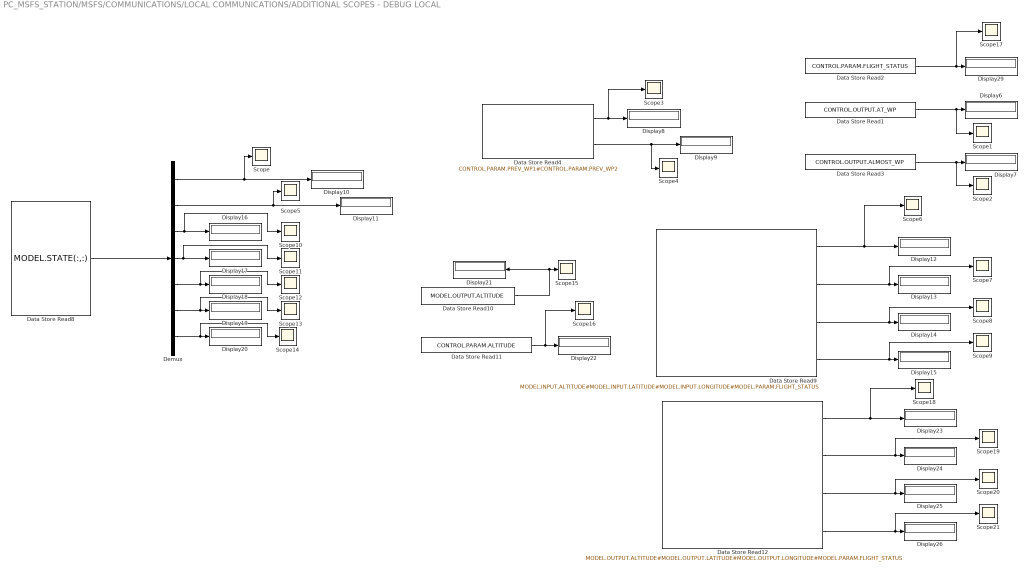
== system PC_MSFS_STATION/MSFS/COMMUNICATIONS/LOCAL COMMUNICATIONS/ADDITIONAL SCOPES - DEBUG LOCAL ==
  Data Store Read1 : DataStoreRead  DataStoreName=CONTROL  DataStoreElements=CONTROL.OUTPUT.AT_WP  IndexOptions=Index vector (dialog)  Indices=1  OutputSizes=1
  Data Store Read10 : DataStoreRead  DataStoreName=MODEL  DataStoreElements=MODEL.OUTPUT.ALTITUDE  IndexOptions=Index vector (dialog)  Indices=1  OutputSizes=1
  Data Store Read11 : DataStoreRead  DataStoreName=CONTROL  DataStoreElements=CONTROL.PARAM.ALTITUDE  IndexOptions=Index vector (dialog)  Indices=1  OutputSizes=1
  Data Store Read12 : DataStoreRead  DataStoreName=MODEL  DataStoreElements=MODEL.OUTPUT.ALTITUDE#MODEL.OUTPUT.LATITUDE#MODEL.OUTPUT.LONGITUDE#MODEL.PARAM.FLIGHT_STATUS  IndexOptions=Index vector (dialog)  Indices=1  OutputSizes=1
  Data Store Read2 : DataStoreRead  DataStoreName=CONTROL  DataStoreElements=CONTROL.PARAM.FLIGHT_STATUS  IndexOptions=Index vector (dialog)  Indices=1  OutputSizes=1
  Data Store Read3 : DataStoreRead  DataStoreName=CONTROL  DataStoreElements=CONTROL.OUTPUT.ALMOST_WP  IndexOptions=Index vector (dialog)  Indices=1  OutputSizes=1
  Data Store Read4 : DataStoreRead  DataStoreName=CONTROL  DataStoreElements=CONTROL.PARAM.PREV_WP1#CONTROL.PARAM.PREV_WP2  IndexOptions=Index vector (dialog)  Indices=1  OutputSizes=1
  Data Store Read8 : DataStoreRead  DataStoreName=MODEL  SampleTime=MODEL_INI.PARAM.SIM_SAMPLING_TIME  DataStoreElements=MODEL.STATE(:,:)  IndexOptions=Index vector (dialog)  Indices=1  OutputSizes=1
  Data Store Read9 : DataStoreRead  DataStoreName=MODEL  DataStoreElements=MODEL.INPUT.ALTITUDE#MODEL.INPUT.LATITUDE#MODEL.INPUT.LONGITUDE#MODEL.PARAM.FLIGHT_STATUS  IndexOptions=Index vector (dialog)  Indices=1  OutputSizes=1
  Demux : Demux  Outputs=7
  Display{6..26,29} (22 alike) : Display
  Scope{,1..21} (22 alike) : Scope
  wires:
  Demux/4 -> Scope11/1, Display17/1
  Data Store Read4/1 -> Scope3/1, Display8/1
  Data Store Read9/3 -> Scope8/1, Display14/1
  Data Store Read11/1 -> Scope16/1, Display22/1
  Data Store Read9/2 -> Scope7/1, Display13/1
  Demux/7 -> Scope14/1, Display20/1
  Data Store Read4/2 -> Scope4/1, Display9/1
  Data Store Read10/1 -> Display21/1, Scope15/1
  Data Store Read8/1 -> Demux/1
  Data Store Read2/1 -> Scope17/1, Display29/1
  Demux/5 -> Scope12/1, Display18/1
  Data Store Read12/2 -> Display24/1, Scope19/1
  Demux/3 -> Scope10/1, Display16/1
  Data Store Read9/4 -> Scope9/1, Display15/1
  Demux/6 -> Scope13/1, Display19/1
  Demux/2 -> Scope5/1, Display11/1
  Data Store Read9/1 -> Display12/1, Scope6/1
  Demux/1 -> Scope/1, Display10/1
  Data Store Read1/1 -> Scope1/1, Display6/1
  Data Store Read3/1 -> Scope2/1, Display7/1
  Data Store Read12/1 -> Scope18/1, Display23/1
  Data Store Read12/3 -> Display25/1, Scope20/1
  Data Store Read12/4 -> Display26/1, Scope21/1

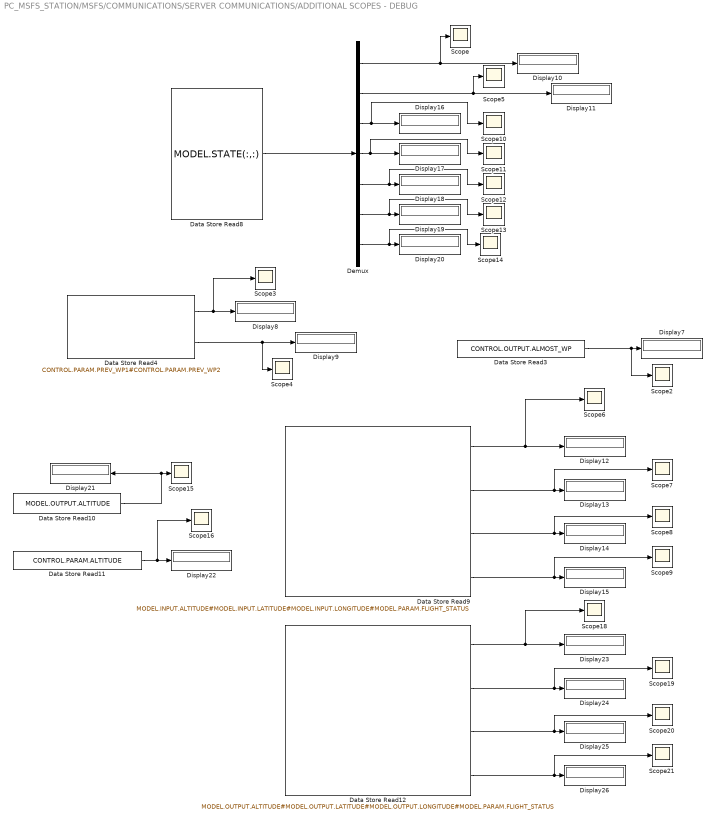
== system PC_MSFS_STATION/MSFS/COMMUNICATIONS/SERVER COMMUNICATIONS/ADDITIONAL SCOPES - DEBUG ==
  Data Store Read10 : DataStoreRead  DataStoreName=MODEL  DataStoreElements=MODEL.OUTPUT.ALTITUDE  IndexOptions=Index vector (dialog)  Indices=1  OutputSizes=1
  Data Store Read11 : DataStoreRead  DataStoreName=CONTROL  DataStoreElements=CONTROL.PARAM.ALTITUDE  IndexOptions=Index vector (dialog)  Indices=1  OutputSizes=1
  Data Store Read12 : DataStoreRead  DataStoreName=MODEL  DataStoreElements=MODEL.OUTPUT.ALTITUDE#MODEL.OUTPUT.LATITUDE#MODEL.OUTPUT.LONGITUDE#MODEL.PARAM.FLIGHT_STATUS  IndexOptions=Index vector (dialog)  Indices=1  OutputSizes=1
  Data Store Read3 : DataStoreRead  DataStoreName=CONTROL  DataStoreElements=CONTROL.OUTPUT.ALMOST_WP  IndexOptions=Index vector (dialog)  Indices=1  OutputSizes=1
  Data Store Read4 : DataStoreRead  DataStoreName=CONTROL  DataStoreElements=CONTROL.PARAM.PREV_WP1#CONTROL.PARAM.PREV_WP2  IndexOptions=Index vector (dialog)  Indices=1  OutputSizes=1
  Data Store Read8 : DataStoreRead  DataStoreName=MODEL  SampleTime=MODEL_INI.PARAM.SIM_SAMPLING_TIME  DataStoreElements=MODEL.STATE(:,:)  IndexOptions=Index vector (dialog)  Indices=1  OutputSizes=1
  Data Store Read9 : DataStoreRead  DataStoreName=MODEL  DataStoreElements=MODEL.INPUT.ALTITUDE#MODEL.INPUT.LATITUDE#MODEL.INPUT.LONGITUDE#MODEL.PARAM.FLIGHT_STATUS  IndexOptions=Index vector (dialog)  Indices=1  OutputSizes=1
  Demux : Demux  Outputs=7
  Display{7..26} (20 alike) : Display
  Scope{,2..16,18..21} (20 alike) : Scope
  wires:
  Data Store Read12/4 -> Scope21/1, Display26/1
  Data Store Read4/2 -> Display9/1, Scope4/1
  Data Store Read9/2 -> Display13/1, Scope7/1
  Data Store Read9/1 -> Scope6/1, Display12/1
  Data Store Read3/1 -> Display7/1, Scope2/1
  Demux/4 -> Display17/1, Scope11/1
  Demux/6 -> Display19/1, Scope13/1
  Demux/5 -> Display18/1, Scope12/1
  Data Store Read4/1 -> Display8/1, Scope3/1
  Demux/7 -> Display20/1, Scope14/1
  Data Store Read9/4 -> Display15/1, Scope9/1
  Data Store Read12/3 -> Scope20/1, Display25/1
  Data Store Read8/1 -> Demux/1
  Data Store Read9/3 -> Display14/1, Scope8/1
  Demux/1 -> Display10/1, Scope/1
  Data Store Read10/1 -> Scope15/1, Display21/1
  Data Store Read11/1 -> Display22/1, Scope16/1
  Demux/2 -> Display11/1, Scope5/1
  Demux/3 -> Display16/1, Scope10/1
  Data Store Read12/1 -> Display23/1, Scope18/1
  Data Store Read12/2 -> Scope19/1, Display24/1

== matlab function PC_MSFS_STATION/CONTROL/CONTROL UPDATE ==
  data: CONTROL_IN input; CONTROL output Bus: CONTROL_Bus; STATE input; ALTITUDE_IN input
function CONTROL = CONTROL_UPDATE(CONTROL_IN, STATE, ALTITUDE_IN)
% COPY CONTROL BUS
CONTROL = CONTROL_IN;
CONTROL.PARAM.SIM_TIME = CONTROL.PARAM.SIM_TIME + CONTROL.PARAM.SAMPLING_TIME;
curr_sim_time = CONTROL.PARAM.SIM_TIME;
deltat = CONTROL.PARAM.SAMPLING_TIME;
flight_status = CONTROL.PARAM.FLIGHT_STATUS;
timer = CONTROL.PARAM.TIMER;
sim_control_mode = CONTROL.PARAM.SIM_CONTROL_MODE;
at_wp = CONTROL.OUTPUT.AT_WP;
wp_flag = CONTROL.OUTPUT.ALMOST_WP;
prev_wp1 = CONTROL.PARAM.PREV_WP1;
prev_wp2 = CONTROL.PARAM.PREV_WP2;
%--------------------------------------------------------------------------
% CONTROL PARAMETERS
%--------------------------------------------------------------------------
% Nominal Control Parameters
kyd = CONTROL.PARAM.NAV_D_1;

% Navigation Variables
%altitude = ALTITUDE_IN;
altitude_control = CONTROL.PARAM.ALTITUDE_REF;
%rho = altitude + 20.902e6;

% Extra Parameters
tau_max = CONTROL.PARAM.TAU_MAX;
dist_Goal = CONTROL.PARAM.DIST_GOAL;
%--------------------------------------------------------------------------
% CONTROL TARGETS
%--------------------------------------------------------------------------
simu_end = CONTROL.TARGET.SIMU_END;
target_latitude = CONTROL.TARGET.LATITUDE*pi/180;
target_longitude = CONTROL.TARGET.LONGITUDE*pi/180;
snom = CONTROL.TARGET.VELOCITY;
dist_obstacle = CONTROL.PARAM.DIST_OBSTACLE;
CBF_const = CONTROL.PARAM.CBF_CONST;
%--------------------------------------------------------------------------
% CONTROL OBSTACLES
%--------------------------------------------------------------------------
obs_id = CONTROL.TARGET.OBSTACLE_ID;
obs_lat = CONTROL.TARGET.OBSTACLE_LATITUDE*pi/180;
obs_long = CONTROL.TARGET.OBSTACLE_LONGITUDE*pi/180;
obs_targetclass = CONTROL.TARGET.OBSTACLE_TARGETCLASS; % 1 = AVOID, 0 = FLY OVER
obst_threatclass = CONTROL.TARGET.OBSTACLE_THREATCLASS;
obs_1 = CONTROL.TARGET.OBSTACLE_COORD1;
obs_2 = CONTROL.TARGET.OBSTACLE_COORD2;
%--------------------------------------------------------------------------
% CONTROL CBFS
%--------------------------------------------------------------------------
h = CONTROL.PARAM.CBF_H;
hdot = CONTROL.PARAM.CBF_HDOT;
psi = CONTROL.PARAM.CBF_PSI;
A1_qp = CONTROL.PARAM.CBF_A1QP;
A2_qp = CONTROL.PARAM.CBF_A2QP;
b1_qp = CONTROL.PARAM.CBF_B1QP;
%--------------------------------------------------------------------------
% SYSTEM CURRENT STATE
%--------------------------------------------------------------------------
% Update Current State
y1 = STATE(1);
y2 = STATE(2);
vy1 = STATE(3);
vy2 = STATE(4);

% FLIGHT STATUS 0 = INITIALIZATION
if flight_status == 0
    altitude = ALTITUDE_IN;
    rho = altitude + 20.902e6;
    % VIRTUAL NOMINAL CONTROLLER (tau1, tau2)
    tau1_nom_PD = - kyd*(vy1 - 0);
    tau2_nom_PD = - kyd*(vy2 - 0);
    tau1_applied = tau1_nom_PD;
    tau2_applied = tau2_nom_PD;
    
    if abs(tau1_applied) >= tau_max
        tau1_applied = sign(tau1_applied)*tau_max;
    else
        tau1_applied = tau1_applied;
    end
    
    if abs(tau2_applied) >= tau_max
        tau2_applied = sign(tau2_applied)*tau_max;
    else
        tau2_applied = tau2_applied;
    end
    if curr_sim_time >= 5
        flight_status = 1;
        timer = 0;
    end 

elseif flight_status == 1
    altitude = altitude_control;
    rho = altitude + 20.902e6;
    tau1_nom_PD = - kyd*(vy1 - 0);
    tau2_nom_PD = - kyd*(vy2 - 0);
    tau1_applied = tau1_nom_PD;
    tau2_applied = tau2_nom_PD;
    
    if abs(tau1_applied) >= tau_max
        tau1_applied = sign(tau1_applied)*tau_max;
    else
        tau1_applied = tau1_applied;
    end
    
    if abs(tau2_applied) >= tau_max
        tau2_applied = sign(tau2_applied)*tau_max;
    else
        tau2_applied = tau2_applied;
    end
    if curr_sim_time >= 8
        flight_status = 2;
        timer = 0;
    end
else
    % ON FLIGHT
    %--------------------------------------------------------------------------
    % DERIVATIVE (D) CONTROL
    %--------------------------------------------------------------------------
    altitude = altitude_control;
    rho = altitude + 20.902e6; 
    timer = timer + deltat;

    wp1 = rho*cos(target_latitude)*cos(target_longitude);
    wp2 = rho*cos(target_latitude)*sin(target_longitude);
    
    if (timer < 2*deltat)
        prev_wp1 = wp1;
        prev_wp2 = wp2;
        CONTROL.PARAM.PREV_WP1 = wp1;
        CONTROL.PARAM.PREV_WP2 = wp2;
    end

    % NOMINAL CONTROLLER
    % System Quadrant
    pos1_PD = wp1 - y1;
    pos2_PD = wp2 - y2;

    if pos1_PD >=0
        % First or fourth quadrant
        if pos2_PD >=0
            %First quadrant
            theta_PD = atan(abs(pos2_PD)/abs(pos1_PD));
        else
            % Fourth quadrant
            %                 theta_PD = 2*pi - atan(abs(pos2_PD)/abs(pos1_PD));
            theta_PD = - atan(abs(pos2_PD)/abs(pos1_PD));
        end
    else
        % Second or third quadrant
        if pos2_PD >=0
            % Second quadrant
            theta_PD = pi - atan(abs(pos2_PD)/abs(pos1_PD));
        else
            % Third quadrant
            theta_PD = pi + atan(abs(pos2_PD)/abs(pos1_PD));
        end
    end

    % New target velocity
    vs1_PD = snom*cos(theta_PD);
    vs2_PD = snom*sin(theta_PD);

    % VIRTUAL NOMINAL CONTROLLER (tau1, tau2)
    tau1_nom_PD = - kyd*(vy1 - vs1_PD);
    tau2_nom_PD = - kyd*(vy2 - vs2_PD);

    if sim_control_mode == 0
        %------------------------------------------------------------------
        % TRACKING ONLY
        %------------------------------------------------------------------
        tau1_applied = tau1_nom_PD;
        tau2_applied = tau2_nom_PD;
    else
        %------------------------------------------------------------------
        % CBF - SAFETY FILTERS: Multiple Obstacles
        %------------------------------------------------------------------
        for i = 1:1:length(obs_id)
            if (obs_id(i) > 0)
                obs_1(i) = rho*cos(obs_lat(i))*cos(obs_long(i));
                obs_2(i) = rho*cos(obs_lat(i))*sin(obs_long(i));

                if (obs_targetclass(i) == 1)
                    dist_obs_scaled = obst_threatclass(i)*dist_obstacle;
                    h(i) = (y1 - obs_1(i))^2 + (y2 - obs_2(i))^2 - dist_obs_scaled^2;
                    hdot(i) = 2*(y1 - obs_1(i))*vy1 + 2*(y2 - obs_2(i))*vy2;
                    psi(i) = hdot(i) + CBF_const*h(i);
                    A1_qp(i) = 2*(y1 - obs_1(i));
                    A2_qp(i) = 2*(y2 - obs_2(i));
                    b1_qp(i) = 2*(vy1^2 + vy2^2) + CBF_const*hdot(i) + CBF_const*psi(i);
                else
                    h(i) = 0;
                    hdot(i) = 0;
                    psi(i) = 0;
                    A1_qp(i) = 0;
                    A2_qp(i) = 0;
                    b1_qp(i) = 0;
                end
            end
        end

        A_qp = -[A1_qp(:), A2_qp(:)];
        b_qp = [b1_qp(:)];
        H_qp = 2*[1, 0; 0, 1];
        f_qp = -2*[tau1_nom_PD; tau2_nom_PD];
        x0_qp = [tau1_nom_PD; tau2_nom_PD];
        option_qp = optimoptions('quadprog','Algorithm','active-set','Display','None');
        [tau_applied, fval_qp, exitval_qp] = quadprog(H_qp, double(f_qp), A_qp, b_qp,[],[],[],[],x0_qp,option_qp);
        tau1_applied = tau_applied(1);
        tau2_applied = tau_applied(2);

        CONTROL.PARAM.CBF_H = h(:);
        CONTROL.PARAM.CBF_PSI = psi(:);
    end


    if abs(tau1_applied) >= tau_max
        tau1_applied = sign(tau1_applied)*tau_max;
    else
        tau1_applied = tau1_applied;
    end

    if abs(tau2_applied) >= tau_max
        tau2_applied = sign(tau2_applied)*tau_max;
    else
        tau2_applied = tau2_applied;
    end
    
    % UPDATE WP FLAG
    if (((y1 - wp1)^2 < (10*100*dist_Goal)^2)&&((y2 - wp2)^2 < (10*100*dist_Goal)^2))
%     if ((y1 - wp1)^2 + (y2 - wp2)^2 < (1000*dist_Goal)^2)
        wp_flag = 1;
    end
    
    % UPDATE TARGET WAYPOINT
    if ((y1 - wp1)^2 + (y2 - wp2)^2 < dist_Goal^2)
        at_wp = 1;
        CONTROL.PARAM.PREV_WP1 = wp1;
        CONTROL.PARAM.PREV_WP2 = wp2;
    end

    if ((prev_wp1 ~= wp1)||(prev_wp2 ~= wp2))
        at_wp = 0;
        wp_flag = 0;
    end
end


%%%%%%%%%%%%%%%%%%%%%%%%%%%%%%%%%%%%%%%%%%%%%%%%%%%%%%%%%%%%%%%%%%%%%%%%%%%
% OUTPUT BUS
%%%%%%%%%%%%%%%%%%%%%%%%%%%%%%%%%%%%%%%%%%%%%%%%%%%%%%%%%%%%%%%%%%%%%%%%%%%
CONTROL.TARGET.SIMU_END = simu_end;
CONTROL.OUTPUT.TAU1 = tau1_applied;
CONTROL.OUTPUT.TAU2 = tau2_applied;

CONTROL.OUTPUT.TAU1_NOM = tau1_nom_PD;
CONTROL.OUTPUT.TAU2_NOM = tau2_nom_PD;

CONTROL.PARAM.FLIGHT_STATUS = flight_status;
CONTROL.PARAM.ALTITUDE = altitude;
CONTROL.PARAM.RHO = rho;
CONTROL.PARAM.TIMER = timer;

CONTROL.OUTPUT.AT_WP = at_wp;
CONTROL.OUTPUT.ALMOST_WP = wp_flag;

return
